simulink model "EKF_slopeestimation"  (R2019b)
settings: Solver=VariableStepAuto  StartTime=0.0  StopTime=4.0  FixedStep=0.05  RelTol=1e-3
settings Model: Creator=win10  LastModifiedBy=win10

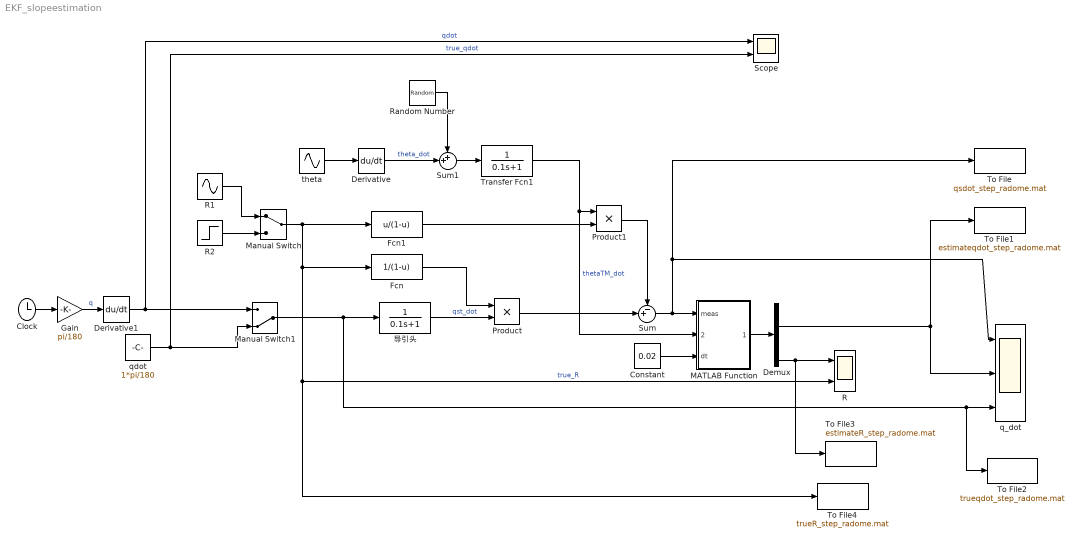
== system EKF_slopeestimation ==
  Clock : Clock
  Constant : Constant  Value=0.02
  Demux : Demux
  Derivative : Derivative
  Derivative1 : Derivative
  Fcn : Fcn  Expr=1/(1-u)
  Fcn1 : Fcn  Expr=u/(1-u)
  Gain : Gain  Gain=pi/180
  MATLAB Function : MATLAB Function  TreatAsAtomicUnit=on
  Manual Switch : ManualSwitch
  Manual Switch1 : ManualSwitch  CurrentSetting=0
  Product : Product
  Product1 : Product
  R : Scope  NumInputPorts=2
  R1 : Sin  Amplitude=0.06  Frequency=pi  SampleTime=0
  R2 : Step  Time=2  Before=0.06  After=0.03  SampleTime=0
  Random Number : RandomNumber  Variance=0.04*pi*pi/180/180  SampleTime=0.1
  Scope : Scope  NumInputPorts=2
  Sum : Sum  Inputs=-+|
  Sum1 : Sum  Inputs=++|
  To File : ToFile  Filename=qsdot_step_radome.mat  MatrixName=qsdot_step_radome
  To File1 : ToFile  Filename=estimateqdot_step_radome.mat  MatrixName=estimateqdot_step_radome
  To File2 : ToFile  Filename=trueqdot_step_radome.mat  MatrixName=trueqdot_step_radome
  To File3 : ToFile  Filename=estimateR_step_radome.mat  MatrixName=estimateR_step_radome
  To File4 : ToFile  Filename=trueR_step_radome.mat  MatrixName=trueR_step_radome
  Transfer Fcn1 : TransferFcn  Denominator=[0.1 1]
  q_dot : Scope  NumInputPorts=3
  qdot : Constant  Value=1*pi/180
  theta : Sin  Amplitude=3*pi/180  Frequency=4*pi  SampleTime=0
  导引头 : TransferFcn  Denominator=[0.1 1]
  wires:
  导引头/1 -> Product/2  "qst_dot"
  Fcn/1 -> Product/1
  Product/1 -> Sum/2
  Sum1/1 -> Transfer Fcn1/1
  Random Number/1 -> Sum1/1
  Fcn1/1 -> Product1/2
  Transfer Fcn1/1 -> MATLAB Function/2(thetaTM_dot), Product1/1  "thetaTM_dot"
  Product1/1 -> Sum/1
  Derivative/1 -> Sum1/2  "theta_dot"
  theta/1 -> Derivative/1
  Sum/1 -> To File/1, q_dot/1, MATLAB Function/1(meas)
  MATLAB Function/1(xhatOut) -> Demux/1
  Demux/4 -> To File3/1, R/1
  R2/1 -> Manual Switch/2
  R1/1 -> Manual Switch/1
  Manual Switch/1 -> To File4/1, R/2, Fcn/1, Fcn1/1  "true_R"
  Derivative1/1 -> Manual Switch1/1, Scope/1  "qdot"
  qdot/1 -> Manual Switch1/2, Scope/2  "true_qdot"
  Gain/1 -> Derivative1/1  "q"
  Clock/1 -> Gain/1
  Constant/1 -> MATLAB Function/3(dt)
  Manual Switch1/1 -> To File2/1, q_dot/3, 导引头/1
  Demux/2 -> To File1/1, q_dot/2

== matlab function EKF_slopeestimation/MATLAB Function ==
  settings: updateMethod=DISCRETE  sampleTime=0.02
  data: meas input; xhatOut output; thetaTM_dot input; dt input
function xhatOut = ExtKalman_Simulink(meas,thetaTM_dot,dt)
% This Embedded MATLAB Function implements an extended Kalman filter used
% for target tracking.
%
% The continuous-time process model is given by
% dx/dt = A*x + B*w

% where, x = [q q_dot qst_dot rou]', q,q_dot is true LOS angle and LOS rate 
% qst_dot is true output of LOS rate from seeker, rou is the radome error
% slope. w = [0 w2 0  w4]'

% Discretize the LTI system model.
%x_k+1 = D*x_k + E*w_k

% and the measurements are given by
% y = qst_dot/(1-rou) - rou/(1-rou)*thetaTM_dot

% Define storage for the variables that need to persist
% between time periods.
Td = 0.1;

persistent P xhat Q R
if isempty(P)
% First time through the code so do some initialization
 xhat = [0;0;0;0];
 P = diag([1 1 1 0.005]);
 Q = diag([0 1e-5/dt 0 1e-3/dt]);
 R = diag([0.04*pi*pi/180/180]);
end


% Calculate the Jacobians for the state equations
% Dynamic state transition matrix in continous-time domain.
A = [0 1 0 0;
     0 0 0 0;
     0 1/Td -1/Td 0;
     0 0 0 0];
  
% noise matrix in continous-time domain.
B = eye(4);
 
% system matrix in discrete-time domain.
% D = expm(A*dt); 
% E = B*dt;

D = [1 dt 0 0;
     0 1 0 0;
     0 dt/Td 1-dt/Td 0;
     0 0 0 1];
E = [dt 0 0 0;
      0 dt 0 0;
      0 0 dt 0;
      0 0 0 dt];
  
% Propogate the state and covariance matrices
xhat = D*xhat;
% xhat = xhat + A*xhat*dt;
P = D*P*D' + E*Q*E';
  
% Calculate the Jacobians for the measurement equations
   q = xhat(1);
   q_dot = xhat(2);
   qst_dot = xhat(3);  
   rou = xhat(4);
   
yhat = qst_dot/(1-rou) - rou/(1-rou)*thetaTM_dot;

H = [0 0 1/(1-rou) (qst_dot-thetaTM_dot)/(1-rou)^2];
    
% Calculate the Kalman gain
K = P*H'/(H*P*H' + R);
% Calculate the measurement residual
resid = meas - yhat;
% Update the state and covariance estimates
xhat = xhat + K*resid;
P = (eye(size(K,1))-K*H)*P;
% Post the results
xhatOut = xhat;


% rangeHat = sqrt(xhat(1)^2+xhat(3)^2);
% bearingHat = atan2(xhat(3),xhat(1));
% yu = [thetaM;psiM];
% yhat = MeasurementModel(xhat);
% H = [cos(bearingHat) 0 sin(bearingHat) 0;
%  -sin(bearingHat)/rangeHat 0 cos(bearingHat)/rangeHat 0];
% % Propogate the state and covariance matrices
% xhat = F*xhat;
% P = F*P*F' + Q;
% % Calculate the Kalman gain
% K = P*H'/(H*P*H' + R);
% % Calculate the measurement residual
% resid = meas - yhat;
% % Update the state and covariance estimates
% xhat = xhat + K*resid;
% P = (eye(size(K,1))-K*H)*P;
% % Post the results
% xhatOut = xhat;
% y = u;
